simulink subsystem "canard_forces_torques"  (R2024b)
settings: Solver=VariableStepAuto  StartTime=0.0  StopTime=10.0  RelTol=1e-3
undefined symbols (not defined in the file or in its folder): canard_area, canard_aspectratio, canard_midchord_angle, canard_pos_x, canard_roll_reversal_factor
settings Model: Creator=trist  LastModifiedBy=finnb

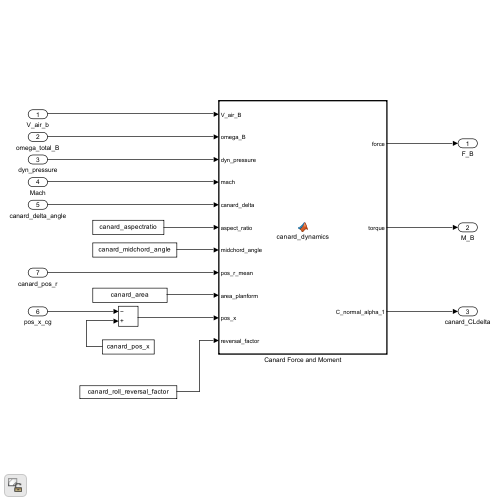
[thumbnail: Simulink's stored preview of the top-level diagram]
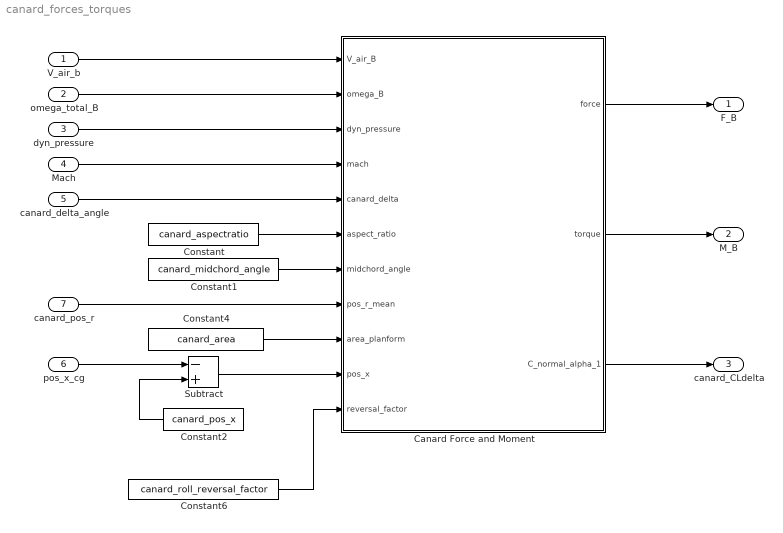
== system canard_forces_torques ==
  V_air_b : Inport
  omega_total_B : Inport  Port=2
  "dyn_pressure " : Inport  Port=3
  "Mach " : Inport  Port=4
  canard_delta_angle : Inport  Port=5
  pos_x_cg : Inport  Port=6
  canard_pos_r : Inport  Port=7
  Canard Force and Moment : MATLAB Function  TreatAsAtomicUnit=on
  Constant : Constant  Value=canard_aspectratio
  Constant1 : Constant  Value=canard_midchord_angle
  Constant2 : Constant  Value=canard_pos_x
  Constant4 : Constant  Value=canard_area
  Constant6 : Constant  Value=canard_roll_reversal_factor
  Subtract : Sum  Inputs=-+
  F_B : Outport  VectorParamsAs1DForOutWhenUnconnected=off
  M_B : Outport  Port=2  VectorParamsAs1DForOutWhenUnconnected=off
  canard_CLdelta : Outport  Port=3  VectorParamsAs1DForOutWhenUnconnected=off
  wires:
  Canard Force and Moment/2(torque) -> M_B/1
  V_air_b/1 -> Canard Force and Moment/1(V_air_B)
  canard_delta_angle/1 -> Canard Force and Moment/5(canard_delta)
  "Mach "/1 -> Canard Force and Moment/4(mach)
  "dyn_pressure "/1 -> Canard Force and Moment/3(dyn_pressure)
  Canard Force and Moment/3(C_normal_alpha_1) -> canard_CLdelta/1
  omega_total_B/1 -> Canard Force and Moment/2(omega_B)
  Constant/1 -> Canard Force and Moment/6(aspect_ratio)
  Constant1/1 -> Canard Force and Moment/7(midchord_angle)
  canard_pos_r/1 -> Canard Force and Moment/8(pos_r_mean)
  Constant4/1 -> Canard Force and Moment/9(area_planform)
  Constant2/1 -> Subtract/2
  pos_x_cg/1 -> Subtract/1
  Subtract/1 -> Canard Force and Moment/10(pos_x)
  Constant6/1 -> Canard Force and Moment/11(reversal_factor)
  Canard Force and Moment/1(force) -> F_B/1

== matlab function canard_forces_torques/Canard Force and Moment ==
  data: force output; V_air_B input; omega_B input; dyn_pressure input; mach input; canard_delta input; aspect_ratio input; midchord_angle input; pos_r_mean input; area_planform input; pos_x input; torque output; C_normal_alpha_1 output; reversal_factor input
function [force, torque, C_normal_alpha_1] = canard_dynamics(V_air_B, omega_B, dyn_pressure, mach, canard_delta, aspect_ratio, midchord_angle, pos_r_mean, area_planform, pos_x, reversal_factor)
    % canard position
    pos = [pos_x; pos_r_mean; 0];

    % relative velocity
    Vrel = V_air_B + cross(omega_B, pos);
    
    % local incidence 
    alpha_local = atan2(Vrel(3), Vrel(1));
    incidence = canard_delta - alpha_local;
    
    % calculate coefficient of planar surface
    C_normal_alpha_1 = aerosurface_online(mach, incidence, aspect_ratio, midchord_angle) * reversal_factor;
    
    % force and torque
    force = C_normal_alpha_1 * area_planform * incidence * dyn_pressure * [0; 0; 1];
    torque = cross(pos, force);
end
